simulink model "Tq_comb_TSD"  (R2022b)
settings: Solver=daessc  StartTime=0.0  StopTime=2.5  RelTol=1e-3
InitFcn:
  | %% Tq_comb_TSD.slx
  | % InitFcn
  | %
  | spring_stiffness = 1e7;
  | viscous_friction_coeff = 10;
  | current_limit = 12.5;
  | %
  | torque_start_t = 1;
  | torque_fin_val = -45; % N M
  | %
  | inertia_start_t = 2;
  | inertia_init_val = 0.1;
  | inertia_fin_val  = 0.5; % kg m^2
StopFcn:
  | disp(['spring_stiffness was       ' num2str(spring_stiffness)])
  | disp('')
  | disp(['viscous_friction_coeff was ' num2str(viscous_friction_coeff)])
  | disp('')
libraries: fl_lib x67, nesl_utility x36, ee_lib x12, sdl_lib x12, slpidlib x3
(part 2 of 2)

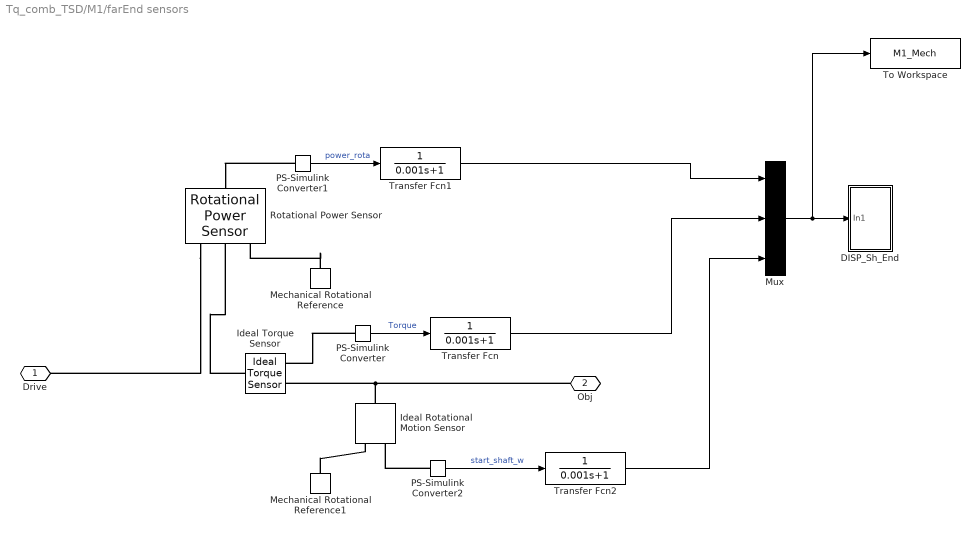
== system Tq_comb_TSD/M1/farEnd sensors ==
  DISP_Sh_End : Subsystem
  Ideal Rotational Motion Sensor : fl_lib/Mechanical/Mechanical Sensors/Ideal Rotational Motion Sensor  reference=foundation.enum.MeasurementReference.difference  acceleration_port=false  velocity_port=true  position_port=false  wrap_angle=false  offset=0 rad
      settings: InternalSimscapePortConfiguration="{\"Bottom\":[],\"Left\":[{\"id\":\"R\",\"label\":\"R\",\"type\":\"foundation.mechanical.rotational.rotational\"}],\"Right\":[{\"id\":\"C\",\"label\":\"C\",\"type\":\"foundation.mechanical.rotational.rotational\"},{\"id\":\"W\",\"label\":\"W\",\"type\":\"output\"}],\"Top\":[]}"
  Ideal Torque Sensor : fl_lib/Mechanical/Mechanical Sensors/Ideal Torque Sensor
  Mechanical Rotational Reference : fl_lib/Mechanical/Rotational Elements/Mechanical Rotational Reference
  Mechanical Rotational Reference1 : fl_lib/Mechanical/Rotational Elements/Mechanical Rotational Reference
  Mux : Mux  Inputs=3
  PS-Simulink Converter : nesl_utility/PS-Simulink Converter  PhysicalDomain=network_engine_domain  SubClassName=ps_output  LeftPortType=input  RightPortType=output  PseudoPeriodic=off  Frequencies=[]  VectorFormat=inherit  Unit=inherit  AffineConversion=off
  PS-Simulink Converter1 : nesl_utility/PS-Simulink Converter  PhysicalDomain=network_engine_domain  SubClassName=ps_output  LeftPortType=input  RightPortType=output  PseudoPeriodic=off  Frequencies=[]  VectorFormat=inherit  Unit=W  AffineConversion=off
  PS-Simulink Converter2 : nesl_utility/PS-Simulink Converter  PhysicalDomain=network_engine_domain  SubClassName=ps_output  LeftPortType=input  RightPortType=output  PseudoPeriodic=off  Frequencies=[]  VectorFormat=inherit  Unit=rpm  AffineConversion=off
  Rotational Power Sensor : sdl_lib/Sensors/Rotational Power Sensor  measurement_type=sdl.enum.rotationalPowerSensorType.instantaneous  averaging_period=1 s  max_frequency=1000 Hz  max_speed=1000 rpm
      settings: InternalSimscapePortConfiguration="{\"Bottom\":[],\"Left\":[{\"id\":\"S\",\"label\":\"S\",\"type\":\"foundation.mechanical.rotational.rotational\"},{\"id\":\"R\",\"label\":\"R\",\"type\":\"foundation.mechanical.rotational.rotational\"},{\"id\":\"C\",\"label\":\"C\",\"type\":\"foundation.mechanical.rotational.rotational\"}],\"Right\":[{\"id\":\"P\",\"label\":\"P\",\"type\":\"output\"}],\"Top\":[]}"
  To Workspace : ToWorkspace  VariableName=M1_Mech  SaveFormat=Timeseries  SampleTime=-1
  Transfer Fcn : TransferFcn  Denominator=[0.001 1]
  Transfer Fcn1 : TransferFcn  Denominator=[0.001 1]
  Transfer Fcn2 : TransferFcn  Denominator=[0.001 1]
  Drive : PMIOPort  Side=Left
  Obj : PMIOPort  Port=2  Side=Right
  wires:
  PS-Simulink Converter/1 -> Transfer Fcn/1  "Torque"
  PS-Simulink Converter1/1 -> Transfer Fcn1/1  "power_rota"
  PS-Simulink Converter2/1 -> Transfer Fcn2/1  "start_shaft_w"
  Transfer Fcn1/1 -> Mux/1
  Transfer Fcn/1 -> Mux/2
  Transfer Fcn2/1 -> Mux/3
  Mux/1 -> To Workspace/1, DISP_Sh_End/1(In1)
  connections:
  Rotational Power Sensor/LConn1 -- Drive/RConn1
  Obj/RConn1 -- Ideal Rotational Motion Sensor/LConn1 -- Ideal Torque Sensor/RConn1
  PS-Simulink Converter/LConn1 -- Ideal Torque Sensor/RConn2
  Mechanical Rotational Reference/LConn1 -- Rotational Power Sensor/LConn3
  PS-Simulink Converter1/LConn1 -- Rotational Power Sensor/RConn1
  Mechanical Rotational Reference1/LConn1 -- Ideal Rotational Motion Sensor/RConn1
  PS-Simulink Converter2/LConn1 -- Ideal Rotational Motion Sensor/RConn2
  Ideal Torque Sensor/LConn1 -- Rotational Power Sensor/LConn2

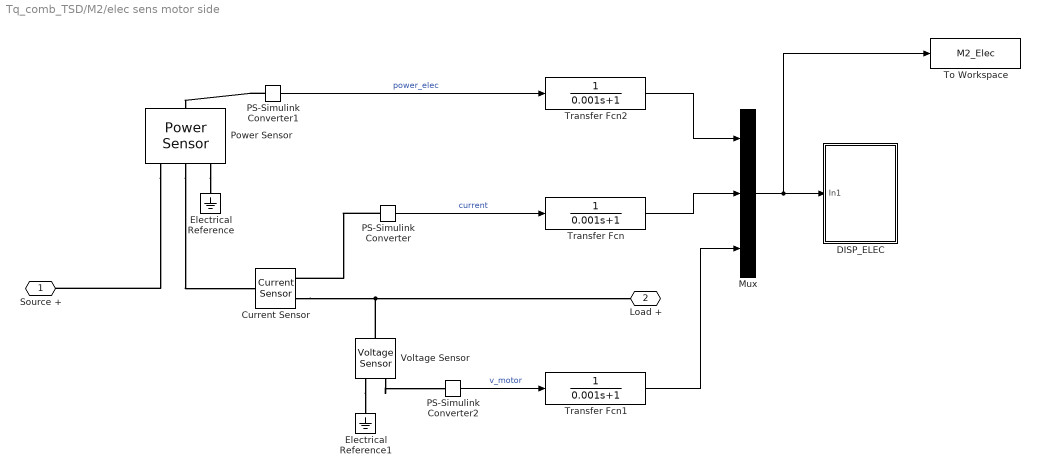
== system Tq_comb_TSD/M2/elec sens motor side ==
  Current Sensor : fl_lib/Electrical/Electrical Sensors/Current Sensor
  DISP_ELEC : Subsystem
  Electrical Reference : fl_lib/Electrical/Electrical Elements/Electrical Reference
  Electrical Reference1 : fl_lib/Electrical/Electrical Elements/Electrical Reference
  Mux : Mux  Inputs=3
  PS-Simulink Converter : nesl_utility/PS-Simulink Converter  PhysicalDomain=network_engine_domain  SubClassName=ps_output  LeftPortType=input  RightPortType=output  PseudoPeriodic=off  Frequencies=[]  VectorFormat=inherit  Unit=A  AffineConversion=off
  PS-Simulink Converter1 : nesl_utility/PS-Simulink Converter  PhysicalDomain=network_engine_domain  SubClassName=ps_output  LeftPortType=input  RightPortType=output  PseudoPeriodic=off  Frequencies=[]  VectorFormat=inherit  Unit=W  AffineConversion=off
  PS-Simulink Converter2 : nesl_utility/PS-Simulink Converter  PhysicalDomain=network_engine_domain  SubClassName=ps_output  LeftPortType=input  RightPortType=output  PseudoPeriodic=off  Frequencies=[]  VectorFormat=inherit  Unit=V  AffineConversion=off
  Power Sensor : ee_lib/Sensors & Transducers/Power Sensor  measurement_type=1  averaging_period=1e-4 s
  To Workspace : ToWorkspace  VariableName=M2_Elec  SaveFormat=Timeseries  SampleTime=-1
  Transfer Fcn : TransferFcn  Denominator=[0.001 1]
  Transfer Fcn1 : TransferFcn  Denominator=[0.001 1]
  Transfer Fcn2 : TransferFcn  Denominator=[0.001 1]
  Voltage Sensor : fl_lib/Electrical/Electrical Sensors/Voltage Sensor
  Source + : PMIOPort  Side=Left
  Load + : PMIOPort  Port=2  Side=Right
  wires:
  Mux/1 -> To Workspace/1, DISP_ELEC/1(In1)
  Transfer Fcn1/1 -> Mux/3
  Transfer Fcn/1 -> Mux/2
  Transfer Fcn2/1 -> Mux/1
  PS-Simulink Converter2/1 -> Transfer Fcn1/1  "v_motor"
  PS-Simulink Converter1/1 -> Transfer Fcn2/1  "power_elec"
  PS-Simulink Converter/1 -> Transfer Fcn/1  "current"
  connections:
  Power Sensor/LConn3 -- Electrical Reference/LConn1
  Power Sensor/LConn2 -- Current Sensor/LConn1
  Voltage Sensor/RConn1 -- PS-Simulink Converter2/LConn1
  Voltage Sensor/RConn2 -- Electrical Reference1/LConn1
  PS-Simulink Converter1/LConn1 -- Power Sensor/RConn1
  PS-Simulink Converter/LConn1 -- Current Sensor/RConn1
  Voltage Sensor/LConn1 -- Load +/RConn1 -- Current Sensor/RConn2
  Power Sensor/LConn1 -- Source +/RConn1

== system Tq_comb_TSD/M2/elec sens v source ==
  Current Sensor : fl_lib/Electrical/Electrical Sensors/Current Sensor
  DISP_ELEC : Subsystem
  Electrical Reference : fl_lib/Electrical/Electrical Elements/Electrical Reference
  Electrical Reference1 : fl_lib/Electrical/Electrical Elements/Electrical Reference
  Mux : Mux  Inputs=3
  PS-Simulink Converter : nesl_utility/PS-Simulink Converter  PhysicalDomain=network_engine_domain  SubClassName=ps_output  LeftPortType=input  RightPortType=output  PseudoPeriodic=off  Frequencies=[]  VectorFormat=inherit  Unit=A  AffineConversion=off
  PS-Simulink Converter1 : nesl_utility/PS-Simulink Converter  PhysicalDomain=network_engine_domain  SubClassName=ps_output  LeftPortType=input  RightPortType=output  PseudoPeriodic=off  Frequencies=[]  VectorFormat=inherit  Unit=W  AffineConversion=off
  PS-Simulink Converter2 : nesl_utility/PS-Simulink Converter  PhysicalDomain=network_engine_domain  SubClassName=ps_output  LeftPortType=input  RightPortType=output  PseudoPeriodic=off  Frequencies=[]  VectorFormat=inherit  Unit=V  AffineConversion=off
  Power Sensor : ee_lib/Sensors & Transducers/Power Sensor  measurement_type=1  averaging_period=1e-4 s
  Transfer Fcn : TransferFcn  Denominator=[0.001 1]
  Transfer Fcn1 : TransferFcn  Denominator=[0.001 1]
  Transfer Fcn2 : TransferFcn  Denominator=[0.001 1]
  Voltage Sensor : fl_lib/Electrical/Electrical Sensors/Voltage Sensor
  Source + : PMIOPort  Side=Left
  Load + : PMIOPort  Port=2  Side=Right
  wires:
  PS-Simulink Converter/1 -> Transfer Fcn/1  "current"
  PS-Simulink Converter1/1 -> Transfer Fcn2/1  "power_elec"
  PS-Simulink Converter2/1 -> Transfer Fcn1/1  "v_motor"
  Transfer Fcn2/1 -> Mux/1
  Transfer Fcn/1 -> Mux/2
  Transfer Fcn1/1 -> Mux/3
  Mux/1 -> DISP_ELEC/1(In1)
  connections:
  Power Sensor/LConn1 -- Source +/RConn1
  Current Sensor/RConn2 -- Load +/RConn1 -- Voltage Sensor/LConn1
  PS-Simulink Converter/LConn1 -- Current Sensor/RConn1
  PS-Simulink Converter1/LConn1 -- Power Sensor/RConn1
  Voltage Sensor/RConn2 -- Electrical Reference1/LConn1
  Voltage Sensor/RConn1 -- PS-Simulink Converter2/LConn1
  Power Sensor/LConn2 -- Current Sensor/LConn1
  Power Sensor/LConn3 -- Electrical Reference/LConn1

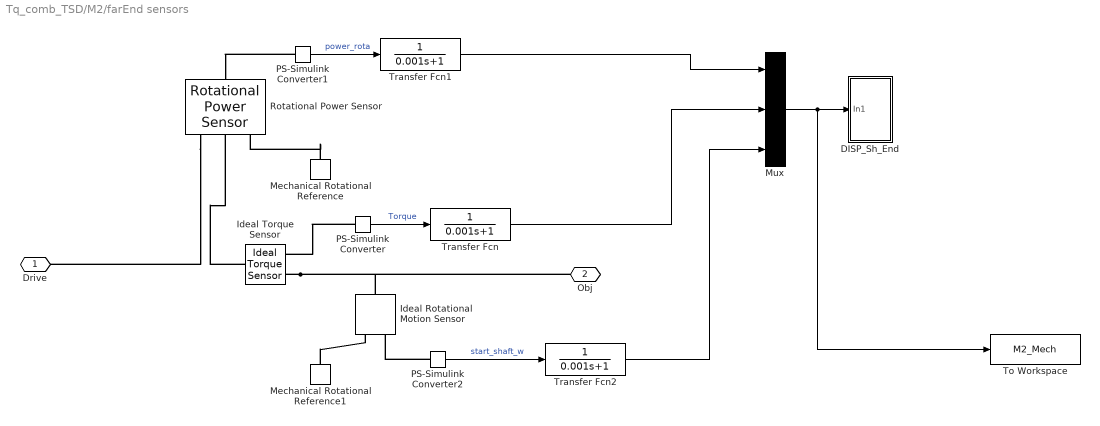
== system Tq_comb_TSD/M2/farEnd sensors ==
  DISP_Sh_End : Subsystem
  Ideal Rotational Motion Sensor : fl_lib/Mechanical/Mechanical Sensors/Ideal Rotational Motion Sensor  reference=foundation.enum.MeasurementReference.difference  acceleration_port=false  velocity_port=true  position_port=false  wrap_angle=false  offset=0 rad
      settings: InternalSimscapePortConfiguration="{\"Bottom\":[],\"Left\":[{\"id\":\"R\",\"label\":\"R\",\"type\":\"foundation.mechanical.rotational.rotational\"}],\"Right\":[{\"id\":\"C\",\"label\":\"C\",\"type\":\"foundation.mechanical.rotational.rotational\"},{\"id\":\"W\",\"label\":\"W\",\"type\":\"output\"}],\"Top\":[]}"
  Ideal Torque Sensor : fl_lib/Mechanical/Mechanical Sensors/Ideal Torque Sensor
  Mechanical Rotational Reference : fl_lib/Mechanical/Rotational Elements/Mechanical Rotational Reference
  Mechanical Rotational Reference1 : fl_lib/Mechanical/Rotational Elements/Mechanical Rotational Reference
  Mux : Mux  Inputs=3
  PS-Simulink Converter : nesl_utility/PS-Simulink Converter  PhysicalDomain=network_engine_domain  SubClassName=ps_output  LeftPortType=input  RightPortType=output  PseudoPeriodic=off  Frequencies=[]  VectorFormat=inherit  Unit=inherit  AffineConversion=off
  PS-Simulink Converter1 : nesl_utility/PS-Simulink Converter  PhysicalDomain=network_engine_domain  SubClassName=ps_output  LeftPortType=input  RightPortType=output  PseudoPeriodic=off  Frequencies=[]  VectorFormat=inherit  Unit=W  AffineConversion=off
  PS-Simulink Converter2 : nesl_utility/PS-Simulink Converter  PhysicalDomain=network_engine_domain  SubClassName=ps_output  LeftPortType=input  RightPortType=output  PseudoPeriodic=off  Frequencies=[]  VectorFormat=inherit  Unit=rpm  AffineConversion=off
  Rotational Power Sensor : sdl_lib/Sensors/Rotational Power Sensor  measurement_type=sdl.enum.rotationalPowerSensorType.instantaneous  averaging_period=1 s  max_frequency=1000 Hz  max_speed=1000 rpm
      settings: InternalSimscapePortConfiguration="{\"Bottom\":[],\"Left\":[{\"id\":\"S\",\"label\":\"S\",\"type\":\"foundation.mechanical.rotational.rotational\"},{\"id\":\"R\",\"label\":\"R\",\"type\":\"foundation.mechanical.rotational.rotational\"},{\"id\":\"C\",\"label\":\"C\",\"type\":\"foundation.mechanical.rotational.rotational\"}],\"Right\":[{\"id\":\"P\",\"label\":\"P\",\"type\":\"output\"}],\"Top\":[]}"
  To Workspace : ToWorkspace  VariableName=M2_Mech  SaveFormat=Timeseries  SampleTime=-1
  Transfer Fcn : TransferFcn  Denominator=[0.001 1]
  Transfer Fcn1 : TransferFcn  Denominator=[0.001 1]
  Transfer Fcn2 : TransferFcn  Denominator=[0.001 1]
  Drive : PMIOPort  Side=Left
  Obj : PMIOPort  Port=2  Side=Right
  wires:
  Mux/1 -> To Workspace/1, DISP_Sh_End/1(In1)
  Transfer Fcn2/1 -> Mux/3
  Transfer Fcn/1 -> Mux/2
  Transfer Fcn1/1 -> Mux/1
  PS-Simulink Converter2/1 -> Transfer Fcn2/1  "start_shaft_w"
  PS-Simulink Converter1/1 -> Transfer Fcn1/1  "power_rota"
  PS-Simulink Converter/1 -> Transfer Fcn/1  "Torque"
  connections:
  Ideal Torque Sensor/LConn1 -- Rotational Power Sensor/LConn2
  PS-Simulink Converter2/LConn1 -- Ideal Rotational Motion Sensor/RConn2
  Mechanical Rotational Reference1/LConn1 -- Ideal Rotational Motion Sensor/RConn1
  PS-Simulink Converter1/LConn1 -- Rotational Power Sensor/RConn1
  Mechanical Rotational Reference/LConn1 -- Rotational Power Sensor/LConn3
  PS-Simulink Converter/LConn1 -- Ideal Torque Sensor/RConn2
  Ideal Torque Sensor/RConn1 -- Ideal Rotational Motion Sensor/LConn1 -- Obj/RConn1
  Rotational Power Sensor/LConn1 -- Drive/RConn1

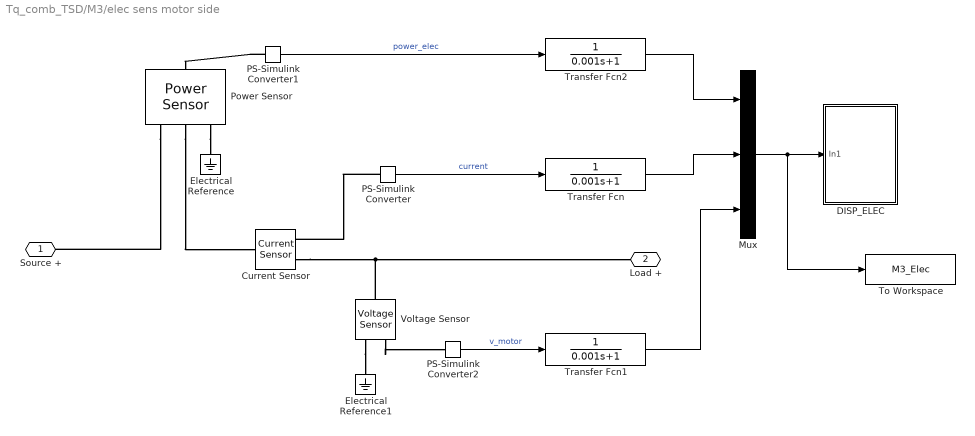
== system Tq_comb_TSD/M3/elec sens motor side ==
  Current Sensor : fl_lib/Electrical/Electrical Sensors/Current Sensor
  DISP_ELEC : Subsystem
  Electrical Reference : fl_lib/Electrical/Electrical Elements/Electrical Reference
  Electrical Reference1 : fl_lib/Electrical/Electrical Elements/Electrical Reference
  Mux : Mux  Inputs=3
  PS-Simulink Converter : nesl_utility/PS-Simulink Converter  PhysicalDomain=network_engine_domain  SubClassName=ps_output  LeftPortType=input  RightPortType=output  PseudoPeriodic=off  Frequencies=[]  VectorFormat=inherit  Unit=A  AffineConversion=off
  PS-Simulink Converter1 : nesl_utility/PS-Simulink Converter  PhysicalDomain=network_engine_domain  SubClassName=ps_output  LeftPortType=input  RightPortType=output  PseudoPeriodic=off  Frequencies=[]  VectorFormat=inherit  Unit=W  AffineConversion=off
  PS-Simulink Converter2 : nesl_utility/PS-Simulink Converter  PhysicalDomain=network_engine_domain  SubClassName=ps_output  LeftPortType=input  RightPortType=output  PseudoPeriodic=off  Frequencies=[]  VectorFormat=inherit  Unit=V  AffineConversion=off
  Power Sensor : ee_lib/Sensors & Transducers/Power Sensor  measurement_type=1  averaging_period=1e-4 s
  To Workspace : ToWorkspace  VariableName=M3_Elec  SaveFormat=Timeseries  SampleTime=-1
  Transfer Fcn : TransferFcn  Denominator=[0.001 1]
  Transfer Fcn1 : TransferFcn  Denominator=[0.001 1]
  Transfer Fcn2 : TransferFcn  Denominator=[0.001 1]
  Voltage Sensor : fl_lib/Electrical/Electrical Sensors/Voltage Sensor
  Source + : PMIOPort  Side=Left
  Load + : PMIOPort  Port=2  Side=Right
  wires:
  PS-Simulink Converter/1 -> Transfer Fcn/1  "current"
  PS-Simulink Converter1/1 -> Transfer Fcn2/1  "power_elec"
  PS-Simulink Converter2/1 -> Transfer Fcn1/1  "v_motor"
  Transfer Fcn2/1 -> Mux/1
  Transfer Fcn/1 -> Mux/2
  Transfer Fcn1/1 -> Mux/3
  Mux/1 -> To Workspace/1, DISP_ELEC/1(In1)
  connections:
  Power Sensor/LConn1 -- Source +/RConn1
  Current Sensor/RConn2 -- Load +/RConn1 -- Voltage Sensor/LConn1
  PS-Simulink Converter/LConn1 -- Current Sensor/RConn1
  PS-Simulink Converter1/LConn1 -- Power Sensor/RConn1
  Voltage Sensor/RConn2 -- Electrical Reference1/LConn1
  Voltage Sensor/RConn1 -- PS-Simulink Converter2/LConn1
  Power Sensor/LConn2 -- Current Sensor/LConn1
  Power Sensor/LConn3 -- Electrical Reference/LConn1

== system Tq_comb_TSD/M3/elec sens v source ==
  Current Sensor : fl_lib/Electrical/Electrical Sensors/Current Sensor
  DISP_ELEC : Subsystem
  Electrical Reference : fl_lib/Electrical/Electrical Elements/Electrical Reference
  Electrical Reference1 : fl_lib/Electrical/Electrical Elements/Electrical Reference
  Mux : Mux  Inputs=3
  PS-Simulink Converter : nesl_utility/PS-Simulink Converter  PhysicalDomain=network_engine_domain  SubClassName=ps_output  LeftPortType=input  RightPortType=output  PseudoPeriodic=off  Frequencies=[]  VectorFormat=inherit  Unit=A  AffineConversion=off
  PS-Simulink Converter1 : nesl_utility/PS-Simulink Converter  PhysicalDomain=network_engine_domain  SubClassName=ps_output  LeftPortType=input  RightPortType=output  PseudoPeriodic=off  Frequencies=[]  VectorFormat=inherit  Unit=W  AffineConversion=off
  PS-Simulink Converter2 : nesl_utility/PS-Simulink Converter  PhysicalDomain=network_engine_domain  SubClassName=ps_output  LeftPortType=input  RightPortType=output  PseudoPeriodic=off  Frequencies=[]  VectorFormat=inherit  Unit=V  AffineConversion=off
  Power Sensor : ee_lib/Sensors & Transducers/Power Sensor  measurement_type=1  averaging_period=1e-4 s
  Transfer Fcn : TransferFcn  Denominator=[0.001 1]
  Transfer Fcn1 : TransferFcn  Denominator=[0.001 1]
  Transfer Fcn2 : TransferFcn  Denominator=[0.001 1]
  Voltage Sensor : fl_lib/Electrical/Electrical Sensors/Voltage Sensor
  Source + : PMIOPort  Side=Left
  Load + : PMIOPort  Port=2  Side=Right
  wires:
  Mux/1 -> DISP_ELEC/1(In1)
  Transfer Fcn1/1 -> Mux/3
  Transfer Fcn/1 -> Mux/2
  Transfer Fcn2/1 -> Mux/1
  PS-Simulink Converter2/1 -> Transfer Fcn1/1  "v_motor"
  PS-Simulink Converter1/1 -> Transfer Fcn2/1  "power_elec"
  PS-Simulink Converter/1 -> Transfer Fcn/1  "current"
  connections:
  Power Sensor/LConn3 -- Electrical Reference/LConn1
  Power Sensor/LConn2 -- Current Sensor/LConn1
  Voltage Sensor/RConn1 -- PS-Simulink Converter2/LConn1
  Voltage Sensor/RConn2 -- Electrical Reference1/LConn1
  PS-Simulink Converter1/LConn1 -- Power Sensor/RConn1
  PS-Simulink Converter/LConn1 -- Current Sensor/RConn1
  Voltage Sensor/LConn1 -- Load +/RConn1 -- Current Sensor/RConn2
  Power Sensor/LConn1 -- Source +/RConn1

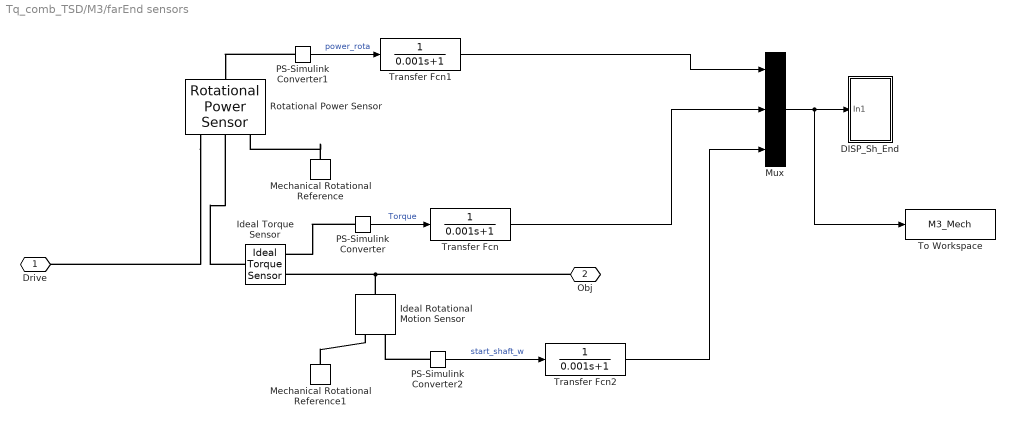
== system Tq_comb_TSD/M3/farEnd sensors ==
  DISP_Sh_End : Subsystem
  Ideal Rotational Motion Sensor : fl_lib/Mechanical/Mechanical Sensors/Ideal Rotational Motion Sensor  reference=foundation.enum.MeasurementReference.difference  acceleration_port=false  velocity_port=true  position_port=false  wrap_angle=false  offset=0 rad
      settings: InternalSimscapePortConfiguration="{\"Bottom\":[],\"Left\":[{\"id\":\"R\",\"label\":\"R\",\"type\":\"foundation.mechanical.rotational.rotational\"}],\"Right\":[{\"id\":\"C\",\"label\":\"C\",\"type\":\"foundation.mechanical.rotational.rotational\"},{\"id\":\"W\",\"label\":\"W\",\"type\":\"output\"}],\"Top\":[]}"
  Ideal Torque Sensor : fl_lib/Mechanical/Mechanical Sensors/Ideal Torque Sensor
  Mechanical Rotational Reference : fl_lib/Mechanical/Rotational Elements/Mechanical Rotational Reference
  Mechanical Rotational Reference1 : fl_lib/Mechanical/Rotational Elements/Mechanical Rotational Reference
  Mux : Mux  Inputs=3
  PS-Simulink Converter : nesl_utility/PS-Simulink Converter  PhysicalDomain=network_engine_domain  SubClassName=ps_output  LeftPortType=input  RightPortType=output  PseudoPeriodic=off  Frequencies=[]  VectorFormat=inherit  Unit=inherit  AffineConversion=off
  PS-Simulink Converter1 : nesl_utility/PS-Simulink Converter  PhysicalDomain=network_engine_domain  SubClassName=ps_output  LeftPortType=input  RightPortType=output  PseudoPeriodic=off  Frequencies=[]  VectorFormat=inherit  Unit=W  AffineConversion=off
  PS-Simulink Converter2 : nesl_utility/PS-Simulink Converter  PhysicalDomain=network_engine_domain  SubClassName=ps_output  LeftPortType=input  RightPortType=output  PseudoPeriodic=off  Frequencies=[]  VectorFormat=inherit  Unit=rpm  AffineConversion=off
  Rotational Power Sensor : sdl_lib/Sensors/Rotational Power Sensor  measurement_type=sdl.enum.rotationalPowerSensorType.instantaneous  averaging_period=1 s  max_frequency=1000 Hz  max_speed=1000 rpm
      settings: InternalSimscapePortConfiguration="{\"Bottom\":[],\"Left\":[{\"id\":\"S\",\"label\":\"S\",\"type\":\"foundation.mechanical.rotational.rotational\"},{\"id\":\"R\",\"label\":\"R\",\"type\":\"foundation.mechanical.rotational.rotational\"},{\"id\":\"C\",\"label\":\"C\",\"type\":\"foundation.mechanical.rotational.rotational\"}],\"Right\":[{\"id\":\"P\",\"label\":\"P\",\"type\":\"output\"}],\"Top\":[]}"
  To Workspace : ToWorkspace  VariableName=M3_Mech  SaveFormat=Timeseries  SampleTime=-1
  Transfer Fcn : TransferFcn  Denominator=[0.001 1]
  Transfer Fcn1 : TransferFcn  Denominator=[0.001 1]
  Transfer Fcn2 : TransferFcn  Denominator=[0.001 1]
  Drive : PMIOPort  Side=Left
  Obj : PMIOPort  Port=2  Side=Right
  wires:
  PS-Simulink Converter/1 -> Transfer Fcn/1  "Torque"
  PS-Simulink Converter1/1 -> Transfer Fcn1/1  "power_rota"
  PS-Simulink Converter2/1 -> Transfer Fcn2/1  "start_shaft_w"
  Transfer Fcn1/1 -> Mux/1
  Transfer Fcn/1 -> Mux/2
  Transfer Fcn2/1 -> Mux/3
  Mux/1 -> To Workspace/1, DISP_Sh_End/1(In1)
  connections:
  Rotational Power Sensor/LConn1 -- Drive/RConn1
  Obj/RConn1 -- Ideal Rotational Motion Sensor/LConn1 -- Ideal Torque Sensor/RConn1
  PS-Simulink Converter/LConn1 -- Ideal Torque Sensor/RConn2
  Mechanical Rotational Reference/LConn1 -- Rotational Power Sensor/LConn3
  PS-Simulink Converter1/LConn1 -- Rotational Power Sensor/RConn1
  Mechanical Rotational Reference1/LConn1 -- Ideal Rotational Motion Sensor/RConn1
  PS-Simulink Converter2/LConn1 -- Ideal Rotational Motion Sensor/RConn2
  Ideal Torque Sensor/LConn1 -- Rotational Power Sensor/LConn2

== system Tq_comb_TSD/M1/elec sens motor side/DISP_ELEC ==
  In1 : Inport
  Demux : Demux  Outputs=3
  tag scope: current_M1=global, power_elec_M1=global, v_motor_M1=global
  wires:
  Demux/2 -> [current_M1]
  Demux/1 -> [power_elec_M1]
  Demux/3 -> [v_motor_M1]
  In1/1 -> Demux/1

== system Tq_comb_TSD/M1/elec sens v source/DISP_ELEC ==
  In1 : Inport
  Demux : Demux  Outputs=3
  Terminator1 : Terminator
  tag scope: curr_in_M1=global, v_in_M1=global
  wires:
  In1/1 -> Demux/1
  Demux/3 -> [v_in_M1]
  Demux/1 -> Terminator1/1
  Demux/2 -> [curr_in_M1]

== system Tq_comb_TSD/M1/farEnd sensors/DISP_Sh_End ==
  In1 : Inport
  Demux : Demux  Outputs=3
  tag scope: Speed_M1=global, power_rota_M1=global, torque_M1=global
  wires:
  In1/1 -> Demux/1
  Demux/1 -> [power_rota_M1]
  Demux/2 -> [torque_M1]
  Demux/3 -> [Speed_M1]

== system Tq_comb_TSD/M2/elec sens motor side/DISP_ELEC ==
  In1 : Inport
  Demux : Demux  Outputs=3
  tag scope: current_M2=global, power_elec_M2=global, v_motor_M2=global
  wires:
  In1/1 -> Demux/1
  Demux/3 -> [v_motor_M2]
  Demux/1 -> [power_elec_M2]
  Demux/2 -> [current_M2]

== system Tq_comb_TSD/M2/elec sens v source/DISP_ELEC ==
  In1 : Inport
  Demux : Demux  Outputs=3
  Terminator : Terminator
  Terminator1 : Terminator
  tag scope: v_in_M2=global
  wires:
  Demux/2 -> Terminator/1
  Demux/1 -> Terminator1/1
  Demux/3 -> [v_in_M2]
  In1/1 -> Demux/1

== system Tq_comb_TSD/M2/farEnd sensors/DISP_Sh_End ==
  In1 : Inport
  Demux : Demux  Outputs=3
  tag scope: Speed_M2=global, power_rota_M2=global, torque_M2=global
  wires:
  Demux/3 -> [Speed_M2]
  Demux/2 -> [torque_M2]
  Demux/1 -> [power_rota_M2]
  In1/1 -> Demux/1

== system Tq_comb_TSD/M3/elec sens motor side/DISP_ELEC ==
  In1 : Inport
  Demux : Demux  Outputs=3
  tag scope: current_M3=global, power_elec_M3=global, v_motor_M3=global
  wires:
  Demux/2 -> [current_M3]
  Demux/1 -> [power_elec_M3]
  Demux/3 -> [v_motor_M3]
  In1/1 -> Demux/1

== system Tq_comb_TSD/M3/elec sens v source/DISP_ELEC ==
  In1 : Inport
  Demux : Demux  Outputs=3
  Terminator : Terminator
  Terminator1 : Terminator
  tag scope: v_in_M3=global
  wires:
  In1/1 -> Demux/1
  Demux/3 -> [v_in_M3]
  Demux/1 -> Terminator1/1
  Demux/2 -> Terminator/1

== system Tq_comb_TSD/M3/farEnd sensors/DISP_Sh_End ==
  In1 : Inport
  Demux : Demux  Outputs=3
  tag scope: Speed_M3=global, power_rota_M3=global, torque_M3=global
  wires:
  In1/1 -> Demux/1
  Demux/1 -> [power_rota_M3]
  Demux/2 -> [torque_M3]
  Demux/3 -> [Speed_M3]
